simulink model "PID Controller"  (R2020b)
settings: Solver=VariableStepAuto  StartTime=0.0  StopTime=500  RelTol=1e-3
undefined symbols (not defined in the file): A, B, C, D
libraries: simulink x1, pid_lib x1
settings Model: Creator=rohan  LastModifiedBy=rohan

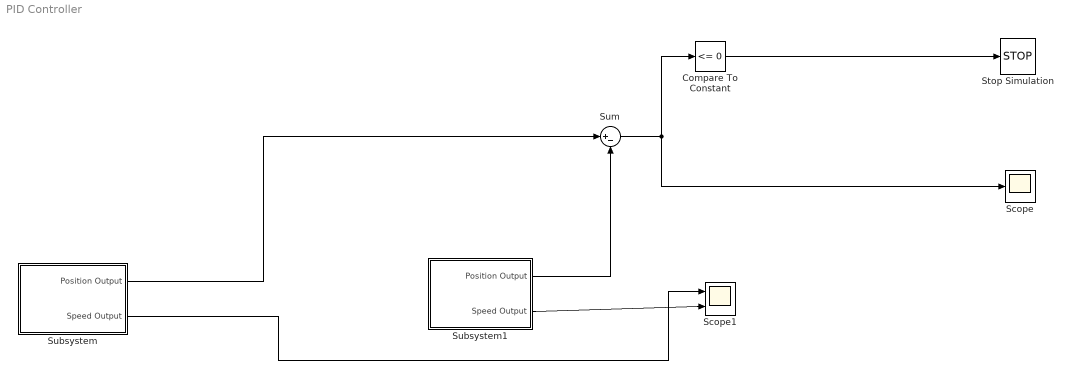
== system PID Controller ==
  Compare To Constant : simulink/Logic and Bit Operations/Compare To Constant  relop=<=  const=0  OutDataTypeStr=boolean
  Scope : Scope
  Scope1 : Scope  NumInputPorts=2
  Stop Simulation : Stop
  Subsystem : Subsystem
  Subsystem1 : Subsystem
  Sum : Sum  Inputs=|+-
  wires:
  Compare To Constant/1 -> Stop Simulation/1
  Sum/1 -> Compare To Constant/1, Scope/1
  Subsystem/1(Position Output) -> Sum/1
  Subsystem1/1(Position Output) -> Sum/2
  Subsystem/2(Speed Output) -> Scope1/1
  Subsystem1/2(Speed Output) -> Scope1/2

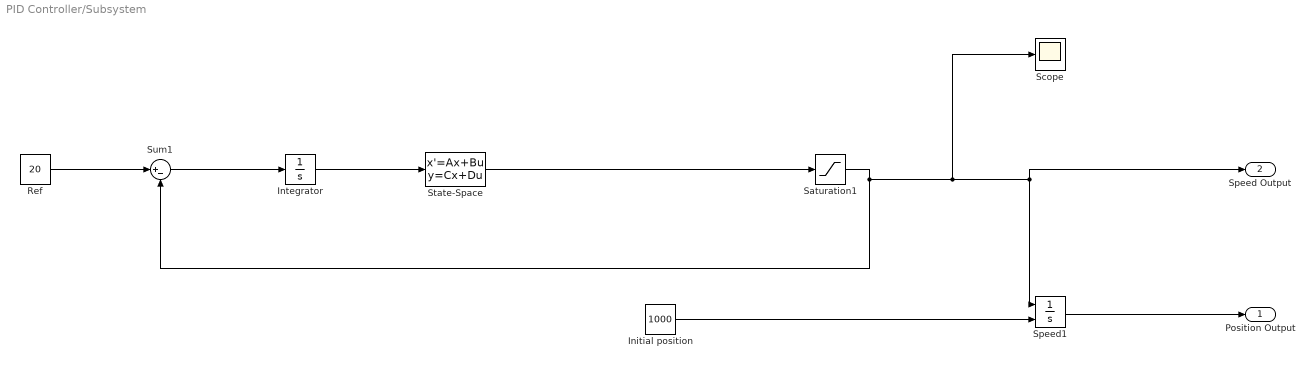
== system PID Controller/Subsystem ==
  Initial position : Constant  Value=1000
  Integrator : Integrator
  Ref : Constant  Value=20
  Saturation1 : Saturate  UpperLimit=40  LowerLimit=0
  Scope : Scope
  Speed1 : Integrator  InitialConditionSource=external
  State-Space : StateSpace  A=A  B=B  C=C  D=D  InitialCondition=25
  Sum1 : Sum  Inputs=|+-
  Position Output : Outport
  Speed Output : Outport  Port=2
  wires:
  Ref/1 -> Sum1/1
  Saturation1/1 -> Sum1/2, Scope/1, Speed Output/1, Speed1/1
  Sum1/1 -> Integrator/1
  State-Space/1 -> Saturation1/1
  Speed1/1 -> Position Output/1
  Initial position/1 -> Speed1/2
  Integrator/1 -> State-Space/1

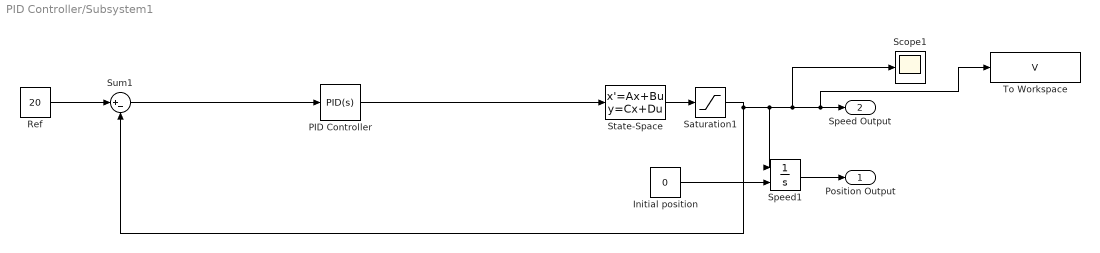
== system PID Controller/Subsystem1 ==
  Initial position : Constant  Value=0
  PID Controller : pid_lib/PID Controller  Controller=PID  Form=Parallel  TimeDomain=Continuous-time  UseExternalTs=off  SampleTime=-1  IntegratorMethod=Forward Euler  FilterMethod=Forward Euler  ControllerParametersSource=internal  P=27.7593  I=3.9352  D=24.0508  UseFilter=on  N=100  TunerSelectOption=Transfer Function Based (PID Tuner App)  InitialConditionSource=internal  InitialConditionForIntegrator=0  InitialConditionForFilter=0  DifferentiatorICPrevScaledInput=0  ExternalReset=none  TrackingMode=off  Kt=1  LimitOutput=off  SatLimitsSource=internal  UpperSaturationLimit=inf  LowerSaturationLimit=-inf  LinearizeAsGain=on  AntiWindupMode=none  Kb=1  POutMin=[]  POutMax=[]  IOutMin=[]  IOutMax=[]  DOutMin=[]  DOutMax=[]  NOutMin=[]  NOutMax=[]  SumOutMin=[]  SumOutMax=[]  SaturationOutMin=[]  SaturationOutMax=[]  PParamMin=[]  PParamMax=[]  IParamMin=[]  IParamMax=[]  DParamMin=[]  DParamMax=[]  NParamMin=[]  NParamMax=[]  KbParamMin=[]  KbParamMax=[]  KtParamMin=[]  KtParamMax=[]  KbOutMin=[]  KbOutMax=[]  KtOutMin=[]  KtOutMax=[]  IntegratorOutMin=[]  IntegratorOutMax=[]  FilterOutMin=[]  FilterOutMax=[]  SumI1OutMin=[]  SumI1OutMax=[]  SumI2OutMin=[]  SumI2OutMax=[]  SumI3OutMin=[]  SumI3OutMax=[]  SumI4OutMin=[]  SumI4OutMax=[]  SumDOutMin=[]  SumDOutMax=[]  DifferentiatorOutMin=[]  DifferentiatorOutMax=[]  FilterDiffOutCoefMin=[]  FilterDiffOutCoefMax=[]  ReciprocalOutMin=[]  ReciprocalOutMax=[]  SumDenOutMin=[]  SumDenOutMax=[]  SumNumOutMin=[]  SumNumOutMax=[]  DivideOutMin=[]  DivideOutMax=[]  UdiffTsProdOutMin=[]  UdiffTsProdOutMax=[]  NTsProdOutMin=[]  NTsProdOutMax=[]  UintegralTsProdOutMin=[]  UintegralTsProdOutMax=[]  UngainTsProdOutMin=[]  UngainTsProdOutMax=[]  IntegratorContinuousStateAttributes=''  IntegratorStateMustResolveToSignalObject=off  IntegratorRTWStateStorageClass=Auto  FilterContinuousStateAttributes=''  FilterStateMustResolveToSignalObject=off  FilterRTWStateStorageClass=Auto  ParallelPVariant=InternalParameters  IdealPVariant=Disabled  IVariant=InternalParameters  DVariant=InternalParameters  IntegratorVariant=Continuous  SatVariant=Disabled  AWVariant=Passthrough  PCopyVariant=Disabled  TRVariant=Disabled  FdbkBlocksVariant=Forward  IdealPFdbkVariant=Disabled  SatFdbkVariant=Disabled  DerivativeFilterVariant=ContFilter  NVariant=InternalParameters  NCopyVariant=Disabled  FilterICVariant=InternalICsFilter  IntegratorICVariant=InternalICs  ExternalResetVariant=Disabled  TRSumVariant=Passthrough  SumFdbkVariant=Disabled  SumVariant=Sum_PID  TsampFilterVariant=InternalTs  TsampNgainVariant=Passthrough  TsampIntegralVariant=Passthrough  ExternalSaturationOutDataTypeStr=Inherit: Same as second input
  Ref : Constant  Value=20
  Saturation1 : Saturate  UpperLimit=50  LowerLimit=0
  Scope1 : Scope
  Speed1 : Integrator  InitialConditionSource=external
  State-Space : StateSpace  A=A  B=B  C=C  D=0  InitialCondition=40
  Sum1 : Sum  Inputs=|+-
  To Workspace : ToWorkspace  VariableName=V  SaveFormat=Timeseries  SampleTime=1
  Position Output : Outport
  Speed Output : Outport  Port=2
  wires:
  Ref/1 -> Sum1/1
  Speed1/1 -> Position Output/1
  Saturation1/1 -> Sum1/2, Scope1/1, To Workspace/1, Speed Output/1, Speed1/1
  Initial position/1 -> Speed1/2
  Sum1/1 -> PID Controller/1
  State-Space/1 -> Saturation1/1
  PID Controller/1 -> State-Space/1
